simulink model "Motores_ABB"  (R2020b)
settings: Solver=FixedStepAuto  StartTime=0.0  StopTime=10  FixedStep=0.001  RelTol=1e-3
undefined symbols (not defined in the file): X, Y, Z
libraries: sm_lib x57, nesl_utility x16, simulink x5
(part 3 of 3)

== matlab function Motores_ABB/Subsystem/MATLAB Function4 ==
  data: t input; vel output; velmax input; tacel input; tconst input; tdecel input; acel output
function [vel, acel]=trapezoidal(t, velmax, tacel, tconst, tdecel)

%t      = u(1);	% Instante de tiempo actual
%velmax = u(2);  % Velocidad máxima
%tacel  = u(3);	% Tiempo de aceleración
%tconst = u(4);	% Tiempo de velocidad constante
%tdecel = u(5);	% Tiempo de deceleración

% Se calcula la velocidad y la aceleración
if t <= tacel
   % Intervalo de aceleración
   acel = velmax/tacel;
   vel  = acel*t;
else
    if t < (tacel+tconst)
	% Intervalo de velocidad constante
        vel  = velmax;
        acel = 0;
    else
        if t>(tacel+tconst+tdecel)
	   % Velocidad y aceleración nula
           vel  = 0;
           acel = 0;
        else
	   % Intervalo de deceleración
           acel = -velmax/tdecel;
           vel  = velmax+acel*(t-tacel-tconst);
        end         
   end
end

% Se devuelve la velocidad y la aceleración
%VEL = [vel; acel];

== matlab function Motores_ABB/Subsystem/MATLAB Function5 ==
  data: t input; vel output; velmax input; tacel input; tconst input; tdecel input; acel output
function [vel, acel]=trapezoidal(t, velmax, tacel, tconst, tdecel)

%t      = u(1);	% Instante de tiempo actual
%velmax = u(2);  % Velocidad máxima
%tacel  = u(3);	% Tiempo de aceleración
%tconst = u(4);	% Tiempo de velocidad constante
%tdecel = u(5);	% Tiempo de deceleración

% Se calcula la velocidad y la aceleración
if t <= tacel
   % Intervalo de aceleración
   acel = velmax/tacel;
   vel  = acel*t;
else
    if t < (tacel+tconst)
	% Intervalo de velocidad constante
        vel  = velmax;
        acel = 0;
    else
        if t>(tacel+tconst+tdecel)
	   % Velocidad y aceleración nula
           vel  = 0;
           acel = 0;
        else
	   % Intervalo de deceleración
           acel = -velmax/tdecel;
           vel  = velmax+acel*(t-tacel-tconst);
        end         
   end
end

% Se devuelve la velocidad y la aceleración
%VEL = [vel; acel];

== matlab function Motores_ABB/Subsystem/MATLAB Function6 ==
  data: t input; vel output; velmax input; tacel input; tconst input; tdecel input; acel output
function [vel, acel]=trapezoidal(t, velmax, tacel, tconst, tdecel)

%t      = u(1);	% Instante de tiempo actual
%velmax = u(2);  % Velocidad máxima
%tacel  = u(3);	% Tiempo de aceleración
%tconst = u(4);	% Tiempo de velocidad constante
%tdecel = u(5);	% Tiempo de deceleración

% Se calcula la velocidad y la aceleración
if t <= tacel
   % Intervalo de aceleración
   acel = velmax/tacel;
   vel  = acel*t;
else
    if t < (tacel+tconst)
	% Intervalo de velocidad constante
        vel  = velmax;
        acel = 0;
    else
        if t>(tacel+tconst+tdecel)
	   % Velocidad y aceleración nula
           vel  = 0;
           acel = 0;
        else
	   % Intervalo de deceleración
           acel = -velmax/tdecel;
           vel  = velmax+acel*(t-tacel-tconst);
        end         
   end
end

% Se devuelve la velocidad y la aceleración
%VEL = [vel; acel];
